simulink model "xilinx_ssr_8in"  (R2019a)
settings: Solver=VariableStepAuto  StartTime=0.0  StopTime=1024*2  RelTol=1e-3
libraries: xbsIndex_r4 x46, xrbsSSR_Library x8
settings Model: Creator=jpsmith  LastModifiedBy=morag
settings DebuggingCC: ArithmeticOperatorsInVariantConditions=warning

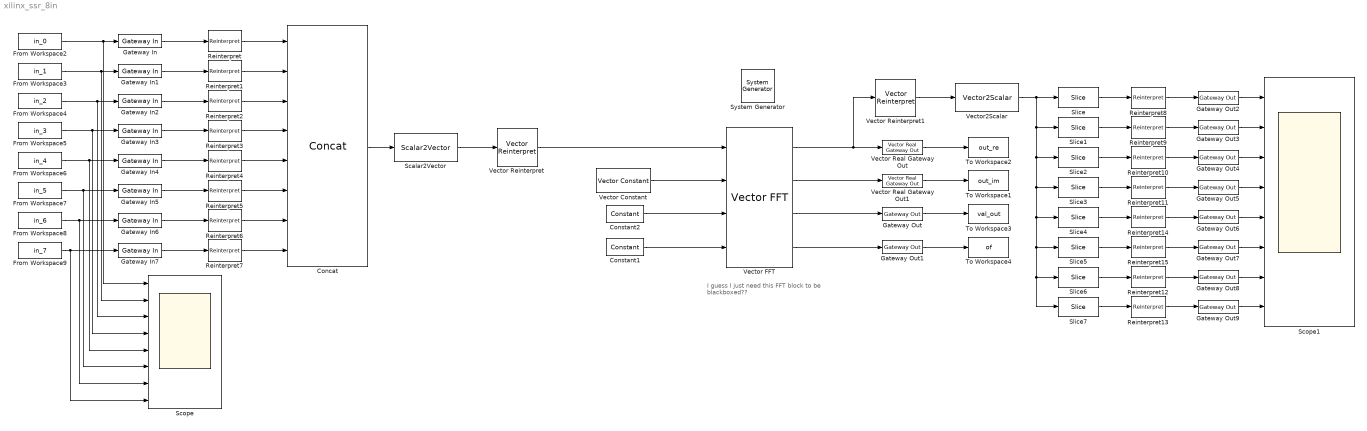
== system xilinx_ssr_8in ==
  note: I guess I just need this FFT block to be blackboxed??
  " System Generator" : xbsIndex_r4/ System Generator  Tag=genX  xilinxfamily=zynquplusRFSOC  part=xczu28dr  speed=-2-e  package=ffvg1517  synthesis_tool=Vivado  clock_wrapper=Clock Enables  directory=./netlist  proj_type=Vivado  Synth_file=Vivado Synthesis Defaults  Impl_file=Vivado Implementation Defaults  testbench=off  simulink_period=1  sysclk_period=10  dcm_input_clock_period=10  incr_netlist=off  trim_vbits=Everywhere in SubSystem  dbl_ovrd=According to Block Masks  core_generation=According to Block Masks  run_coregen=off  deprecated_control=off  eval_field=0  block_type=sysgen
  Concat : xbsIndex_r4/Concat  num_inputs=8  dbl_ovrd=off  block_type=concat
  Constant1 : xbsIndex_r4/Constant  const=0  gui_display_data_type=Fixed-point  arith_type=Signed (2's comp)  n_bits=10  bin_pt=0  preci_type=Single  exp_width=8  frac_width=24  explicit_period=on  period=1  equ=P=C  opselect=C  inp2=PCIN>>17  opr=+  inp1=P  carry=CIN  dbl_ovrd=off  block_type=constant
  Constant2 : xbsIndex_r4/Constant  const=1  gui_display_data_type=Boolean  arith_type=Boolean  n_bits=10  bin_pt=0  preci_type=Single  exp_width=8  frac_width=24  explicit_period=on  period=1  equ=P=C  opselect=C  inp2=PCIN>>17  opr=+  inp1=P  carry=CIN  dbl_ovrd=off  block_type=constant
  From Workspace2 : FromWorkspace  VariableName=in_0  SampleTime=0
  From Workspace3 : FromWorkspace  VariableName=in_1  SampleTime=0
  From Workspace4 : FromWorkspace  VariableName=in_2  SampleTime=0
  From Workspace5 : FromWorkspace  VariableName=in_3  SampleTime=0
  From Workspace6 : FromWorkspace  VariableName=in_4  SampleTime=0
  From Workspace7 : FromWorkspace  VariableName=in_5  SampleTime=0
  From Workspace8 : FromWorkspace  VariableName=in_6  SampleTime=0
  From Workspace9 : FromWorkspace  VariableName=in_7  SampleTime=0
  Gateway In{,1..7} (8 alike) : xbsIndex_r4/Gateway In  gui_display_data_type=Fixed-point  arith_type="Signed  (2's comp)"  n_bits=18  bin_pt=17  preci_type=Single  exp_width=8  frac_width=24  rows=1  columns=1  quantization="Round  (unbiased: +/- Inf)"  overflow=Saturate  period=1  UseAsADC=off  ADCChannel='1'  interface=None  automatic_assignment=on  address_offset=hex2dec('00')  intf_name=''  intf_description=''  default_value=0  timing_constraint=None  locs_specified=off  LOCs={}  io_standard={}  inherit_from_input=off  hdl_port=on  dbl_ovrd=off  block_type=gatewayin
  Gateway Out{,1..9} (10 alike) : xbsIndex_r4/Gateway Out  inherit_from_input=off  hdl_port=on  rows=1  columns=1  UseAsDAC=off  DACChannel='1'  interface=None  automatic_assignment=on  address_offset=hex2dec('00')  intf_name=''  intf_description=''  timing_constraint=None  locs_specified=off  LOCs={}  io_standard={}  block_type=gatewayout
  Reinterpret{,1..7} (8 alike) : xbsIndex_r4/Reinterpret  force_arith_type=on  arith_type=Unsigned  force_bin_pt=on  bin_pt=0  block_type=reinterpret
  Reinterpret{8..15} (8 alike) : xbsIndex_r4/Reinterpret  force_arith_type=on  arith_type="Signed  (2's comp)"  force_bin_pt=on  bin_pt=17  block_type=reinterpret
  Scalar2Vector : xrbsSSR_Library/Scalar2Vector  Width=18  sg_ssr=8  sg_ssr_prev=8  sg_ssr_name=vect_Scalar2Vector  block_type=scalar2vector_ssr
      settings: SourceProductName=Xilinx SSR Blockset
  Scope : Scope  NumInputPorts=8
  Scope1 : Scope  NumInputPorts=8
  Slice : xbsIndex_r4/Slice  nbits=18  boolean_output=off  mode=Upper Bit Location + Width  bit1=0  base1=MSB of Input  bit0=126  base0=LSB of Input  dbl_ovrd=off  block_type=slice
  Slice1 : xbsIndex_r4/Slice  nbits=18  boolean_output=off  mode=Upper Bit Location + Width  bit1=-1*18  base1=MSB of Input  bit0=1  base0=MSB of Input  dbl_ovrd=off  block_type=slice
  Slice2 : xbsIndex_r4/Slice  nbits=18  boolean_output=off  mode=Upper Bit Location + Width  bit1=-2*18  base1=MSB of Input  bit0=126  base0=LSB of Input  dbl_ovrd=off  block_type=slice
  Slice3 : xbsIndex_r4/Slice  nbits=18  boolean_output=off  mode=Upper Bit Location + Width  bit1=-3*18  base1=MSB of Input  bit0=1  base0=MSB of Input  dbl_ovrd=off  block_type=slice
  Slice4 : xbsIndex_r4/Slice  nbits=18  boolean_output=off  mode=Upper Bit Location + Width  bit1=-4*18  base1=MSB of Input  bit0=126  base0=LSB of Input  dbl_ovrd=off  block_type=slice
  Slice5 : xbsIndex_r4/Slice  nbits=18  boolean_output=off  mode=Upper Bit Location + Width  bit1=-5*18  base1=MSB of Input  bit0=1  base0=MSB of Input  dbl_ovrd=off  block_type=slice
  Slice6 : xbsIndex_r4/Slice  nbits=18  boolean_output=off  mode=Upper Bit Location + Width  bit1=-6*18  base1=MSB of Input  bit0=126  base0=LSB of Input  dbl_ovrd=off  block_type=slice
  Slice7 : xbsIndex_r4/Slice  nbits=18  boolean_output=off  mode=Upper Bit Location + Width  bit1=-7*18  base1=MSB of Input  bit0=1  base0=MSB of Input  dbl_ovrd=off  block_type=slice
  To Workspace1 : ToWorkspace  VariableName=out_im  SampleTime=-1
      settings: Save2DSignal=2-D array (concatenate along first dimension)
  To Workspace2 : ToWorkspace  VariableName=out_re  SampleTime=-1
      settings: Save2DSignal=2-D array (concatenate along first dimension)
  To Workspace3 : ToWorkspace  VariableName=val_out  SampleTime=-1
      settings: Save2DSignal=2-D array (concatenate along first dimension)
  To Workspace4 : ToWorkspace  VariableName=of  SampleTime=-1
      settings: Save2DSignal=2-D array (concatenate along first dimension)
  Vector Constant : xrbsSSR_Library/Vector Constant  const=[0,0,0,0,0,0,0,0]  gui_display_data_type=Fixed-point  arith_type=Signed (2's comp)  n_bits=18  bin_pt=17  preci_type=Single  exp_width=8  frac_width=24  explicit_period=off  period=1  sg_ssr=SSR  sg_ssr_prev=8  equ=P=C  opselect=C  inp2=PCIN>>17  opr=+  inp1=P  carry=CIN  dbl_ovrd=off  block_type=constant_ssr
      settings: SourceProductName=Xilinx SSR Blockset
  Vector FFT : xrbsSSR_Library/Vector FFT  sg_ssr=8  N=1024  W_high=1  W_low=-17  n_bits=18  bin_pt=17  bram_threshold=258  block_type=fft_ssr
      settings: SourceProductName=Xilinx SSR Blockset
  Vector Real Gateway Out : xrbsSSR_Library/Vector Real Gateway Out  inherit_from_input=off  hdl_port=on  rows=1  columns=1  UseAsDAC=off  DACChannel='1'  interface=None  automatic_assignment=on  address_offset=hex2dec('00')  intf_name=''  intf_description=''  timing_constraint=None  locs_specified=off  LOCs={}  io_standard={}  block_type=realgatewayout_ssr  sg_ssr=8  sg_ssr_prev=8  sg_ssr_name=vect_real_gwayout
      settings: SourceProductName=Xilinx SSR Blockset  infoedit=The Vector Real Gateway out block converts Xilinx fixed-point or floating-point type vector inputs into vector ouputs of type Simulink integer, single, double, or fixed-point.<br><br>Hardware notes: In hardware these blocks become top level output ports or are discarded, depending on how they are configured.
  Vector Real Gateway Out1 : xrbsSSR_Library/Vector Real Gateway Out  inherit_from_input=off  hdl_port=on  rows=1  columns=1  UseAsDAC=off  DACChannel='1'  interface=None  automatic_assignment=on  address_offset=hex2dec('00')  intf_name=''  intf_description=''  timing_constraint=None  locs_specified=off  LOCs={}  io_standard={}  block_type=realgatewayout_ssr  sg_ssr=8  sg_ssr_prev=8  sg_ssr_name=vect_real_gwayout
      settings: SourceProductName=Xilinx SSR Blockset  infoedit=The Vector Real Gateway out block converts Xilinx fixed-point or floating-point type vector inputs into vector ouputs of type Simulink integer, single, double, or fixed-point.<br><br>Hardware notes: In hardware these blocks become top level output ports or are discarded, depending on how they are configured.
  Vector Reinterpret : xrbsSSR_Library/Vector Reinterpret  sg_ssr=8  sg_ssr_prev=8  force_arith_type=on  arith_type="Signed  (2's comp)"  force_bin_pt=on  bin_pt=17  block_type=reinterpret_ssr
      settings: SourceProductName=Xilinx SSR Blockset  infoedit="The Vector Reinterpret block Changes vector input signal type without altering the binary representation. You can change the signal between signed and unsigned, and relocate the binary point.<br><br>Hardware notes: In hardware this block costs nothing.<br><br>Example:  Suppose the input is 6 bits wide, signed, with 2 fractional bits, and the output is forced to unsigned with 0 fractional bits.  Then an input of -2.0 (1110.00 in binary 2's complement) becomes an output of 56 (111000 in binary)."
  Vector Reinterpret1 : xrbsSSR_Library/Vector Reinterpret  sg_ssr=8  sg_ssr_prev=8  force_arith_type=on  arith_type=Unsigned  force_bin_pt=on  bin_pt=0  block_type=reinterpret_ssr
      settings: SourceProductName=Xilinx SSR Blockset  infoedit="The Vector Reinterpret block Changes vector input signal type without altering the binary representation. You can change the signal between signed and unsigned, and relocate the binary point.<br><br>Hardware notes: In hardware this block costs nothing.<br><br>Example:  Suppose the input is 6 bits wide, signed, with 2 fractional bits, and the output is forced to unsigned with 0 fractional bits.  Then an input of -2.0 (1110.00 in binary 2's complement) becomes an output of 56 (111000 in binary)."
  Vector2Scalar : xrbsSSR_Library/Vector2Scalar  sg_ssr=8  sg_ssr_prev=8  sg_ssr_name=vect_Vector2Scalar  block_type=vector2scalar_ssr
      settings: SourceProductName=Xilinx SSR Blockset
  wires:
  Vector Real Gateway Out/1 -> To Workspace2/1
  Vector Real Gateway Out1/1 -> To Workspace1/1
  Vector Constant/1 -> Vector FFT/2
  Vector FFT/2 -> Vector Real Gateway Out1/1
  Gateway Out1/1 -> To Workspace4/1
  Gateway Out/1 -> To Workspace3/1
  Vector FFT/3 -> Gateway Out/1
  Vector FFT/4 -> Gateway Out1/1
  Constant1/1 -> Vector FFT/4
  Constant2/1 -> Vector FFT/3
  Gateway In7/1 -> Reinterpret7/1
  Gateway In5/1 -> Reinterpret5/1
  Gateway In4/1 -> Reinterpret4/1
  From Workspace3/1 -> Scope/2, Gateway In1/1
  Reinterpret4/1 -> Concat/5
  From Workspace6/1 -> Scope/5, Gateway In4/1
  From Workspace8/1 -> Scope/7, Gateway In6/1
  Scalar2Vector/1 -> Vector Reinterpret/1
  From Workspace9/1 -> Scope/8, Gateway In7/1
  Reinterpret7/1 -> Concat/8
  Reinterpret6/1 -> Concat/7
  From Workspace7/1 -> Scope/6, Gateway In5/1
  Gateway In1/1 -> Reinterpret1/1
  Reinterpret3/1 -> Concat/4
  Reinterpret5/1 -> Concat/6
  Gateway In/1 -> Reinterpret/1
  Reinterpret1/1 -> Concat/2
  Concat/1 -> Scalar2Vector/1
  Reinterpret/1 -> Concat/1
  From Workspace4/1 -> Scope/3, Gateway In2/1
  Reinterpret2/1 -> Concat/3
  Gateway In2/1 -> Reinterpret2/1
  From Workspace2/1 -> Gateway In/1, Scope/1
  From Workspace5/1 -> Scope/4, Gateway In3/1
  Gateway In6/1 -> Reinterpret6/1
  Gateway In3/1 -> Reinterpret3/1
  Vector Reinterpret/1 -> Vector FFT/1
  Vector FFT/1 -> Vector Reinterpret1/1, Vector Real Gateway Out/1
  Vector Reinterpret1/1 -> Vector2Scalar/1
  Vector2Scalar/1 -> Slice2/1, Slice7/1, Slice6/1, Slice5/1, Slice4/1, Slice3/1, Slice1/1, Slice/1
  Gateway Out2/1 -> Scope1/1
  Gateway Out3/1 -> Scope1/2
  Gateway Out4/1 -> Scope1/3
  Gateway Out5/1 -> Scope1/4
  Gateway Out6/1 -> Scope1/5
  Gateway Out7/1 -> Scope1/6
  Gateway Out8/1 -> Scope1/7
  Gateway Out9/1 -> Scope1/8
  Slice/1 -> Reinterpret8/1
  Reinterpret8/1 -> Gateway Out2/1
  Slice1/1 -> Reinterpret9/1
  Reinterpret9/1 -> Gateway Out3/1
  Slice3/1 -> Reinterpret11/1
  Reinterpret11/1 -> Gateway Out5/1
  Slice2/1 -> Reinterpret10/1
  Reinterpret10/1 -> Gateway Out4/1
  Slice6/1 -> Reinterpret12/1
  Reinterpret12/1 -> Gateway Out8/1
  Reinterpret14/1 -> Gateway Out6/1
  Reinterpret13/1 -> Gateway Out9/1
  Slice4/1 -> Reinterpret14/1
  Slice7/1 -> Reinterpret13/1
  Slice5/1 -> Reinterpret15/1
  Reinterpret15/1 -> Gateway Out7/1
